simulink model "simulink_AVP"  (R2016a)
settings: Solver=VariableStepAuto  StartTime=0.0  StopTime=10.0  RelTol=1e-3
undefined symbols (not defined in the file or in its folder): kd, ki, kp
libraries: simulink x1
settings Model: Creator=vipul  LastModifiedBy=vipul

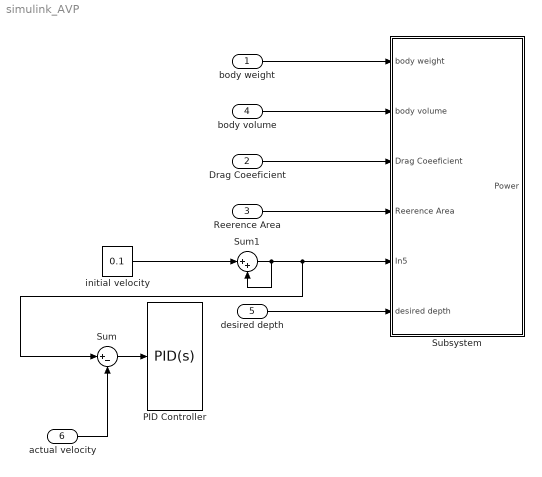
== system simulink_AVP ==
  body weight : Inport
  "Drag Coeeficient " : Inport  Port=2
  Reerence Area : Inport  Port=3
  body volume : Inport  Port=4
  desired depth : Inport  Port=5
  actual velocity : Inport  Port=6
  PID Controller : simulink/Continuous/PID Controller  Controller=PID  TimeDomain=Continuous-time  SampleTime=-1  IntegratorMethod=Forward Euler  FilterMethod=Forward Euler  Form=Parallel  UseFilter=on  ControllerParametersSource=internal  P=kp  I=ki  D=kd  N=100  InitialConditionSource=internal  InitialConditionForIntegrator=0  InitialConditionForFilter=0  ExternalReset=none  LimitOutput=on  UpperSaturationLimit=450  LowerSaturationLimit=-450  LinearizeAsGain=on  AntiWindupMode=none  Kb=1  TrackingMode=off  Kt=1  PParamMin=[]  PParamMax=[]  IParamMin=[]  IParamMax=[]  DParamMin=[]  DParamMax=[]  NParamMin=[]  NParamMax=[]  KbParamMin=[]  KbParamMax=[]  KtParamMin=[]  KtParamMax=[]  POutMin=[]  POutMax=[]  IOutMin=[]  IOutMax=[]  DOutMin=[]  DOutMax=[]  NOutMin=[]  NOutMax=[]  KbOutMin=[]  KbOutMax=[]  KtOutMin=[]  KtOutMax=[]  IntegratorOutMin=[]  IntegratorOutMax=[]  FilterOutMin=[]  FilterOutMax=[]  SumOutMin=[]  SumOutMax=[]  SumI1OutMin=[]  SumI1OutMax=[]  SumI2OutMin=[]  SumI2OutMax=[]  SumI3OutMin=[]  SumI3OutMax=[]  SumDOutMin=[]  SumDOutMax=[]  SaturationOutMin=[]  SaturationOutMax=[]  IntegratorContinuousStateAttributes=''  IntegratorStateMustResolveToSignalObject=off  IntegratorRTWStateStorageClass=Auto  FilterContinuousStateAttributes=''  FilterStateMustResolveToSignalObject=off  FilterRTWStateStorageClass=Auto  DifferentiatorICPrevScaledInput=0  DifferentiatorOutMin=[]  DifferentiatorOutMax=[]
  Subsystem : Subsystem
  Sum : Sum  Inputs=|+-
  Sum1 : Sum  Inputs=|++
  initial velocity : Constant  Value=0.1
  wires:
  Sum1/1 -> Sum1/2, Sum/1, Subsystem/5(In5)
  initial velocity/1 -> Sum1/1
  body weight/1 -> Subsystem/1(body weight)
  body volume/1 -> Subsystem/2(body volume)
  "Drag Coeeficient "/1 -> Subsystem/3("Drag Coeeficient ")
  Reerence Area/1 -> Subsystem/4(Reerence Area)
  desired depth/1 -> Subsystem/6(desired depth)
  Sum/1 -> PID Controller/1
  actual velocity/1 -> Sum/2

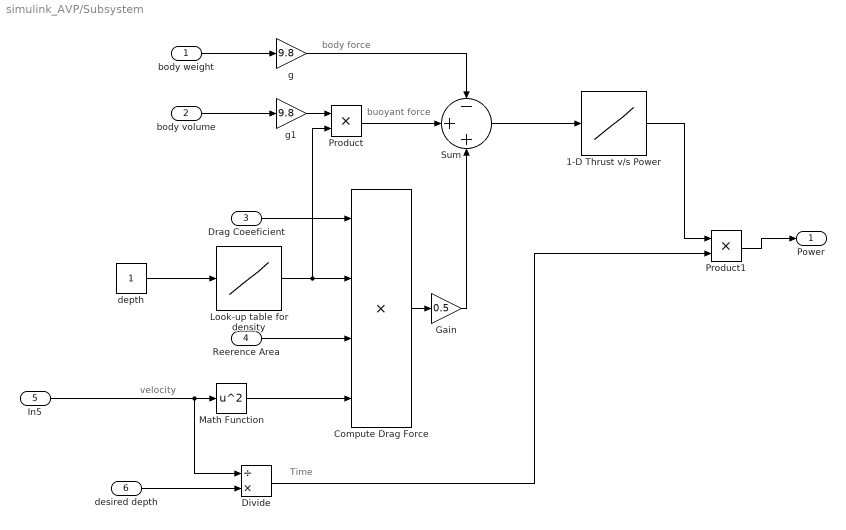
== system simulink_AVP/Subsystem ==
  note: velocity
  note: Time
  note: body force
  note: buoyant force
  body weight : Inport
  body volume : Inport  Port=2
  "Drag Coeeficient " : Inport  Port=3
  Reerence Area : Inport  Port=4
  In5 : Inport  Port=5
  desired depth : Inport  Port=6
  1-D Thrust v/s Power : Lookup_n-D  NumberOfTableDimensions=1  BreakpointsForDimension1=[-5:5]  Table=tanh([-5:5])  InternalRulePriority=Speed  RndMeth=Simplest  InputSameDT=on
  Compute Drag Force : Product  Inputs=4
  Divide : Product  Inputs=/*
  Gain : Gain  Gain=0.5
  Look-up table for density : Lookup_n-D  NumberOfTableDimensions=1  BreakpointsForDimension1=[-5:5]  Table=tanh([-5:5])  InternalRulePriority=Speed  RndMeth=Simplest  InputSameDT=on
  Math Function : Math  Operator=square  SaturateOnIntegerOverflow=on
  Product : Product
  Product1 : Product
  Sum : Sum  Inputs=-++
  depth : Constant
  g : Gain  Gain=9.8
  g1 : Gain  Gain=9.8
  Power : Outport
  wires:
  In5/1 -> Divide/1, Math Function/1
  1-D Thrust v/s Power/1 -> Product1/1
  Product1/1 -> Power/1
  "Drag Coeeficient "/1 -> Compute Drag Force/1
  Gain/1 -> Sum/3
  g1/1 -> Product/1
  Look-up table for density/1 -> Product/2, Compute Drag Force/2
  Reerence Area/1 -> Compute Drag Force/3
  Sum/1 -> 1-D Thrust v/s Power/1
  Divide/1 -> Product1/2
  Compute Drag Force/1 -> Gain/1
  body volume/1 -> g1/1
  g/1 -> Sum/1
  depth/1 -> Look-up table for density/1
  body weight/1 -> g/1
  Product/1 -> Sum/2
  desired depth/1 -> Divide/2
  Math Function/1 -> Compute Drag Force/4
